simulink model "sensors_noise"  (Simulink 7.9)
settings: Solver=ode14x  StartTime=0.0  StopTime=10.0  FixedStep=Tsamp  RelTol=1e-3
values from neighbouring files (symbols this model uses):
  Tsamp = 0.001    [LSDP_controllers_nntraining_data_igva.m]    (also in initialize_LSDP_controllers_igva.m)
  V_b = 1e-15    [Initialise_LQG_observers_igva.m]    (also in LSDP_controllers_nntraining_data_igva.m = 0; initialize_LSDP_controllers_igva.m = 0)
  V_gap = 1e-7    (= 1e-07)    [Initialise_LQG_observers_igva.m]    (also in LSDP_controllers_nntraining_data_igva.m = 0; initialize_LSDP_controllers_igva.m = 0)
  V_i = 1e-7    (= 1e-07)    [Initialise_LQG_observers_igva.m]    (also in LSDP_controllers_nntraining_data_igva.m = 0; initialize_LSDP_controllers_igva.m = 0)
  V_zdot = 1e-7    (= 1e-07)    [Initialise_LQG_observers_igva.m]    (also in initialize_LSDP_controllers_igva.m = 0)
  V_zdotdot = 1e-7    (= 1e-07)    [Initialise_LQG_observers_igva.m]    (also in initialize_LSDP_controllers_igva.m = 0)
libraries: simulink x5
settings Model: Creator=kostas  LastModifiedBy=kostas

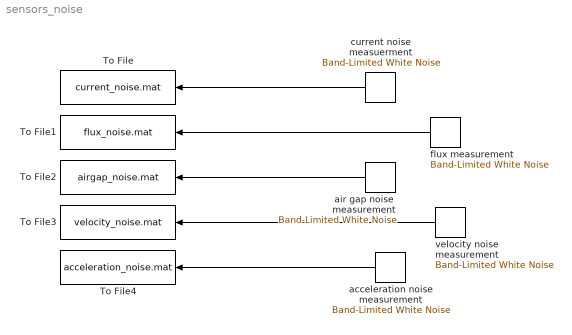
== system sensors_noise ==
  To File : ToFile  Filename=current_noise.mat  MatrixName=current_noise  SaveFormat=Timeseries  SampleTime=Tsamp
  To File1 : ToFile  Filename=flux_noise.mat  MatrixName=flux_noise  SaveFormat=Timeseries  SampleTime=Tsamp
  To File2 : ToFile  Filename=airgap_noise.mat  MatrixName=airgap_noise  SaveFormat=Timeseries  SampleTime=Tsamp
  To File3 : ToFile  Filename=velocity_noise.mat  MatrixName=velocity_noise  SaveFormat=Timeseries  SampleTime=Tsamp
  To File4 : ToFile  Filename=acceleration_noise.mat  MatrixName=acceleration_noise  SaveFormat=Timeseries  SampleTime=Tsamp
  acceleration noise measurement : simulink/Sources/Band-Limited White Noise  Cov=V_zdotdot*Tsamp  Ts=Tsamp  seed=[23341]
  air gap noise  measurement : simulink/Sources/Band-Limited White Noise  Cov=V_gap*Tsamp  Ts=Tsamp  seed=[23356]
  current noise measuerment : simulink/Sources/Band-Limited White Noise  Cov=V_i*Tsamp  Ts=Tsamp  seed=[12331]
  flux measurement : simulink/Sources/Band-Limited White Noise  Cov=V_b*Tsamp  Ts=Tsamp  seed=[21441]
  velocity noise measurement : simulink/Sources/Band-Limited White Noise  Cov=V_zdot*Tsamp  Ts=Tsamp  seed=[22541]
  wires:
  current noise measuerment/1 -> To File/1
  flux measurement/1 -> To File1/1
  air gap noise  measurement/1 -> To File2/1
  velocity noise measurement/1 -> To File3/1
  acceleration noise measurement/1 -> To File4/1
